simulink model "RA_Modes"  (R2022b)
settings: Solver=FixedStepAuto  StartTime=0.0  StopTime=10.0  FixedStep=1e-3  RelTol=1e-3  EnableMultiTasking=on
undefined symbols (not defined in the file): D0, D1, D10, D11, D12, D13, D2, D3, D4, D5, D6, D7, D8, D9, PTA0, PTA1, PTA2, PTB23, PTB9, PTC16, PTC17, PTC2, PTC3, PTC4, PTD0, PTD1, PTD2, PTD3
libraries: frdmk64flib x18, dspstat3 x1
settings Model: ExtModeTrigDuration=5  Creator=sarahalabdulrazzak  LastModifiedBy=kavem
settings SolverCC: AlgebraicLoopSolver=TrustRegion
settings OptimizationCC: EnhancedBackFolding=on  PassReuseOutputArgsAs=Individual arguments  ZeroExternalMemoryAtStartup=off  ZeroInternalMemoryAtStartup=off  MaxStackSize=64  OptimizeBlockOrder=speed  DifferentSizesBufferReuse=on  OptimizationCustomize=off  EfficientTunableParamExpr=on
settings DebuggingCC: ParameterTunabilityLossMsg=error  UnconnectedInputMsg=warning  UnconnectedOutputMsg=warning  UnconnectedLineMsg=warning  SFMachineParentedDataDiag=warning
settings HardwareCC: ProdBitPerPointer=32  ProdBitPerSizeT=32  ProdBitPerPtrDiffT=32  ProdLargestAtomicInteger=Long  ProdLargestAtomicFloat=Double  ProdWordSize=32  ProdHWDeviceType=ARM Compatible->ARM Cortex
settings ModelReferenceCC: EnableRefExpFcnMdlSchedulingChecks=on
settings SFSimCC: MATLABDynamicMemAlloc=off
settings RTWCC: Description=Embedded Coder  SystemTargetFile=ert.tlc  HardwareBoard=NXP FRDM-K64F  TLCOptions="-aInlineSetEventsForThisBaseRateFcn=TLC_FALSE -aSuppressMultiTaskScheduler=TLC_FALSE  -aRateBasedStepFcn=0"  TemplateMakefile=ert_default_tmf  Toolchain=GNU Tools for ARM Embedded Processors
settings CodeAppCC: ForceParamTrailComments=on  IgnoreCustomStorageClasses=off  OperatorAnnotations=on  SimulinkDataObjDesc=on  SFDataObjDesc=on  InsertBlockDesc=on

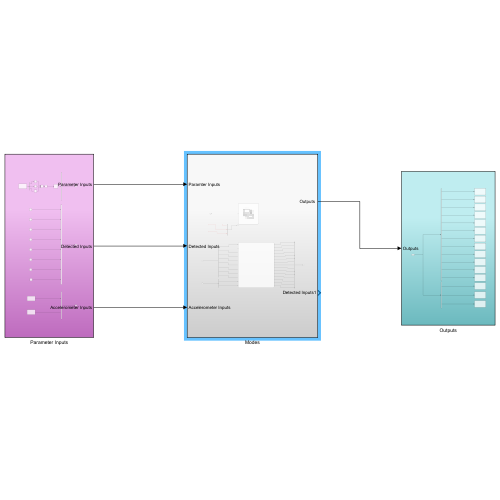
[thumbnail: Simulink's stored preview of the top-level diagram]
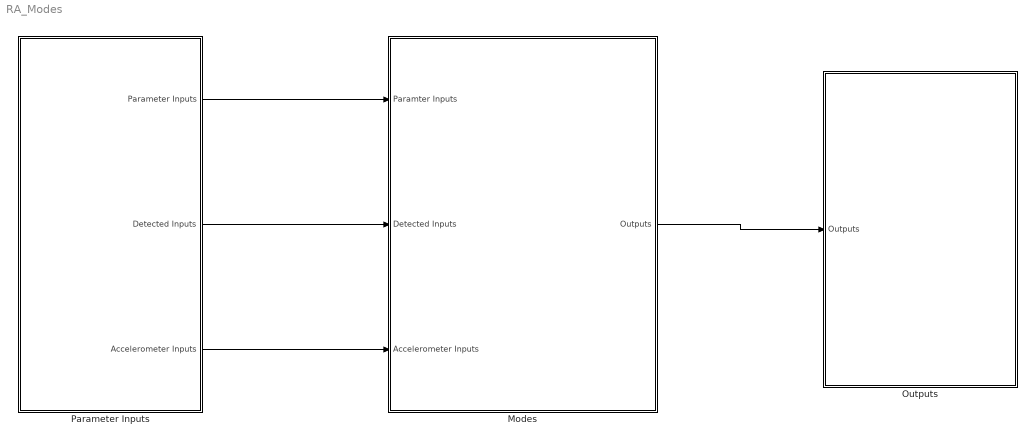
== system RA_Modes ==
  Modes : Subsystem
  Outputs : Subsystem
  Parameter Inputs : Subsystem
  wires:
  Parameter Inputs/1(Parameter Inputs) -> Modes/1(Paramter Inputs)
  Parameter Inputs/2(Detected Inputs) -> Modes/2(Detected Inputs)
  Modes/1("Outputs ") -> Outputs/1("Outputs ")
  Parameter Inputs/3(Accelerometer Inputs) -> Modes/3(Accelerometer Inputs)

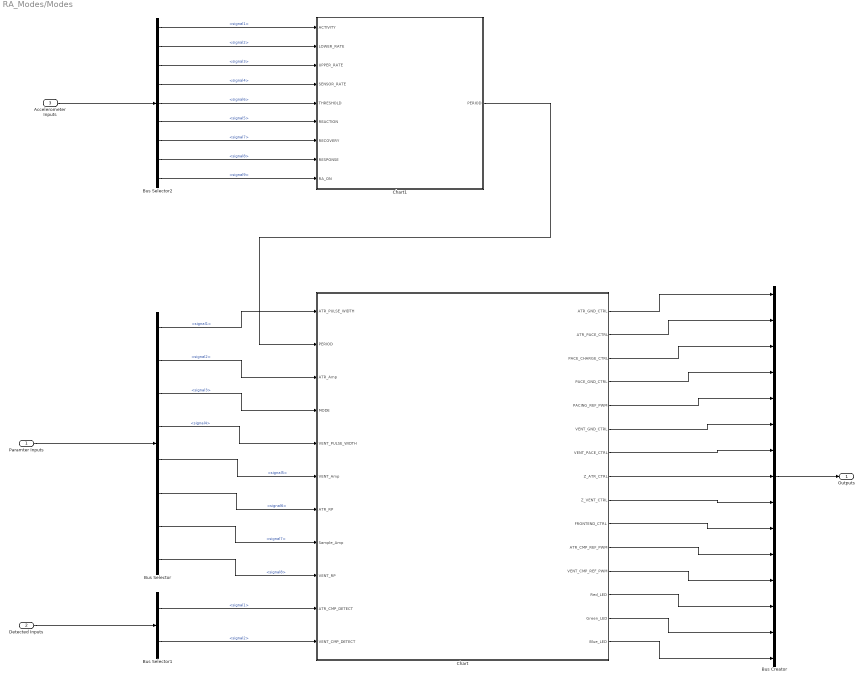
== system RA_Modes/Modes ==
  Paramter Inputs : Inport
  Detected Inputs : Inport  Port=2
  Accelerometer Inputs : Inport  Port=3
  Bus Creator : BusCreator  Inputs=15
  Bus Selector : BusSelector  OutputSignals=signal1,signal2,signal3,signal4,signal5,signal6,signal7,signal8
  Bus Selector1 : BusSelector  OutputSignals=signal1,signal2
  Bus Selector2 : BusSelector  OutputSignals=signal1,signal2,signal3,signal4,signal6,signal5,signal7,signal8,signal9
  Chart : Stateflow chart  TreatAsAtomicUnit=on
  Chart1 : Stateflow chart  TreatAsAtomicUnit=on
  "Outputs " : Outport
  wires:
  Paramter Inputs/1 -> Bus Selector/1
  Detected Inputs/1 -> Bus Selector1/1
  Bus Selector/1 -> Chart/1(ATR_PULSE_WIDTH)  "<signal1>"
  Chart/1(ATR_GND_CTRL) -> Bus Creator/1
  Chart/2(ATR_PACE_CTRL) -> Bus Creator/2
  Chart/4(PACE_GND_CTRL) -> Bus Creator/4
  Chart/5(PACING_REF_PWM) -> Bus Creator/5
  Chart/6(VENT_GND_CTRL) -> Bus Creator/6
  Chart/7(VENT_PACE_CTRL) -> Bus Creator/7
  Chart/8(Z_ATR_CTRL) -> Bus Creator/8
  Chart/9(Z_VENT_CTRL) -> Bus Creator/9
  Chart/10(FRONTEND_CTRL) -> Bus Creator/10
  Chart/11(ATR_CMP_REF_PWM) -> Bus Creator/11
  Chart/12(VENT_CMP_REF_PWM) -> Bus Creator/12
  Bus Creator/1 -> "Outputs "/1
  Chart/14(Green_LED) -> Bus Creator/14
  Chart/15(Blue_LED) -> Bus Creator/15
  Bus Selector1/1 -> Chart/10(ATR_CMP_DETECT)  "<signal1>"
  Bus Selector1/2 -> Chart/11(VENT_CMP_DETECT)  "<signal2>"
  Chart/3(PACE_CHARGE_CTRL) -> Bus Creator/3
  Chart/13(Red_LED) -> Bus Creator/13
  Bus Selector/2 -> Chart/3(ATR_Amp)  "<signal2>"
  Bus Selector/3 -> Chart/4(MODE)  "<signal3>"
  Bus Selector/4 -> Chart/5(VENT_PULSE_WIDTH)  "<signal4>"
  Bus Selector/5 -> Chart/6(VENT_Amp)  "<signal5>"
  Bus Selector/6 -> Chart/7(ATR_RP)  "<signal6>"
  Bus Selector/7 -> Chart/8(Sample_Amp)  "<signal7>"
  Bus Selector/8 -> Chart/9(VENT_RP)  "<signal8>"
  Accelerometer Inputs/1 -> Bus Selector2/1
  Bus Selector2/1 -> Chart1/1(ACTIVITY)  "<signal1>"
  Bus Selector2/2 -> Chart1/2(LOWER_RATE)  "<signal2>"
  Bus Selector2/3 -> Chart1/3(UPPER_RATE)  "<signal3>"
  Bus Selector2/4 -> Chart1/4(SENSOR_RATE)  "<signal4>"
  Bus Selector2/5 -> Chart1/5(THRESHOLD)  "<signal6>"
  Bus Selector2/6 -> Chart1/6(REACTION)  "<signal5>"
  Bus Selector2/7 -> Chart1/7(RECOVERY)  "<signal7>"
  Bus Selector2/8 -> Chart1/8(RESPONSE)  "<signal8>"
  Bus Selector2/9 -> Chart1/9(RA_ON)  "<signal9>"
  Chart1/1(PERIOD) -> Chart/2(PERIOD)

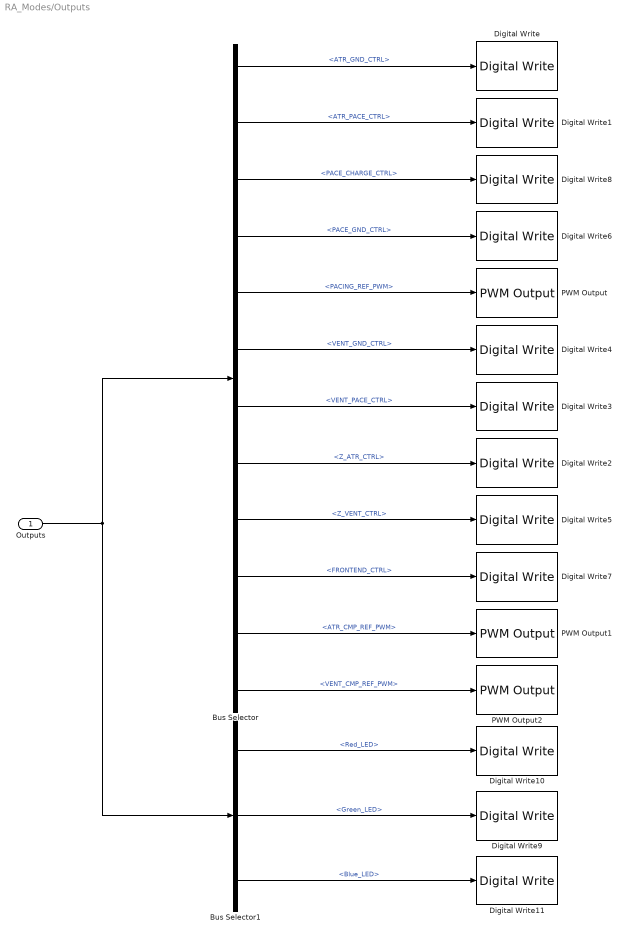
== system RA_Modes/Outputs ==
  "Outputs " : Inport
  Bus Selector : BusSelector  OutputSignals=ATR_GND_CTRL,ATR_PACE_CTRL,PACE_CHARGE_CTRL,PACE_GND_CTRL,PACING_REF_PWM,VENT_GND_CTRL,VENT_PACE_CTRL,Z_ATR_CTRL,Z_VENT_CTRL,FRONTEND_CTRL,ATR_CMP_REF_PWM,VENT_CMP_REF_PWM
  Bus Selector1 : BusSelector  OutputSignals=Red_LED,Green_LED,Blue_LED
  Digital Write : frdmk64flib/Digital Write  Whichpin=PTD2 (D11)
  Digital Write1 : frdmk64flib/Digital Write  Whichpin=PTA0 (D8)
  Digital Write10 : frdmk64flib/Digital Write  Whichpin=RED_LED
  Digital Write11 : frdmk64flib/Digital Write  Whichpin=BLUE_LED
  Digital Write2 : frdmk64flib/Digital Write  Whichpin=PTB23 (D4)
  Digital Write3 : frdmk64flib/Digital Write  Whichpin=PTC4 (D9)
  Digital Write4 : frdmk64flib/Digital Write  Whichpin=PTD3 (D12)
  Digital Write5 : frdmk64flib/Digital Write  Whichpin=PTC3 (D7)
  Digital Write6 : frdmk64flib/Digital Write  Whichpin=PTD0 (D10)
  Digital Write7 : frdmk64flib/Digital Write  Whichpin=PTD1 (D13)
  Digital Write8 : frdmk64flib/Digital Write  Whichpin=PTB9 (D2)
  Digital Write9 : frdmk64flib/Digital Write  Whichpin=GREEN_LED
  PWM Output : frdmk64flib/PWM Output  Whichpin=PTA2 (D5)  InitialFrequency=2000  InitialDutyCycle=0
  PWM Output1 : frdmk64flib/PWM Output  Whichpin=PTC2 (D6)  InitialFrequency=2000  InitialDutyCycle=0
  PWM Output2 : frdmk64flib/PWM Output  Whichpin=PTA1 (D3)  InitialFrequency=2000  InitialDutyCycle=0
  wires:
  Bus Selector/1 -> Digital Write/1  "<ATR_GND_CTRL>"
  Bus Selector/2 -> Digital Write1/1  "<ATR_PACE_CTRL>"
  Bus Selector/3 -> Digital Write8/1  "<PACE_CHARGE_CTRL>"
  Bus Selector/4 -> Digital Write6/1  "<PACE_GND_CTRL>"
  Bus Selector/5 -> PWM Output/1  "<PACING_REF_PWM>"
  Bus Selector/6 -> Digital Write4/1  "<VENT_GND_CTRL>"
  Bus Selector/7 -> Digital Write3/1  "<VENT_PACE_CTRL>"
  Bus Selector/8 -> Digital Write2/1  "<Z_ATR_CTRL>"
  Bus Selector/9 -> Digital Write5/1  "<Z_VENT_CTRL>"
  Bus Selector/10 -> Digital Write7/1  "<FRONTEND_CTRL>"
  Bus Selector/11 -> PWM Output1/1  "<ATR_CMP_REF_PWM>"
  Bus Selector/12 -> PWM Output2/1  "<VENT_CMP_REF_PWM>"
  "Outputs "/1 -> Bus Selector/1, Bus Selector1/1
  Bus Selector1/1 -> Digital Write10/1  "<Red_LED>"
  Bus Selector1/2 -> Digital Write9/1  "<Green_LED>"
  Bus Selector1/3 -> Digital Write11/1  "<Blue_LED>"

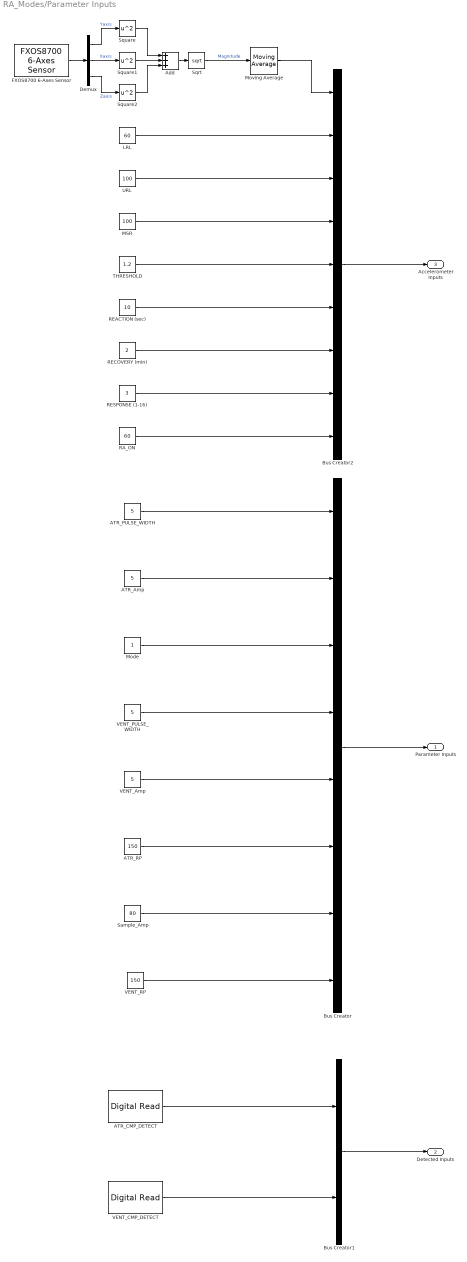
== system RA_Modes/Parameter Inputs ==
  ATR_Amp : Constant  Value=5
  ATR_CMP_DETECT : frdmk64flib/Digital Read  Whichpin=PTC16 (D0)  SampleTime=-1
  ATR_PULSE_WIDTH : Constant  Value=5
  ATR_RP : Constant  Value=150
  Add : Sum  Inputs=+++
  Bus Creator : BusCreator  Inputs=8
  Bus Creator1 : BusCreator  Inputs=2
  Bus Creator2 : BusCreator  Inputs=9
  Demux : Demux  Outputs=3
  FXOS8700 6-Axes Sensor : frdmk64flib/FXOS8700 6-Axes Sensor  Activesensor=Accelerometer only  ODR=800Hz  HybridODR=400Hz  Accelfullrange=-4g to +4g  SampleTime=-1
  LRL : Constant  Value=60
  MSR : Constant  Value=100
  Mode : Constant
  Moving Average : dspstat3/Moving Average  Method=Exponential weighting  ForgettingFactorPort=off  SpecifyWindowLength=on  WindowLength=4  OverlapLength=3  AllowArbitraryInputLength=off  ForgettingFactor=0.999  SimulateUsing=Code generation
  RA_ON : Constant  Value=60
  REACTION (sec) : Constant  Value=10
  RECOVERY (min) : Constant  Value=2
  RESPONSE (1-16) : Constant  Value=3
  Sample_Amp : Constant  Value=80
  Sqrt : Sqrt
  Square : Math  Operator=square
  Square1 : Math  Operator=square
  Square2 : Math  Operator=square
  THRESHOLD : Constant  Value=1.2
  URL : Constant  Value=100
  VENT_Amp : Constant  Value=5
  VENT_CMP_DETECT : frdmk64flib/Digital Read  Whichpin=PTC17 (D1)  SampleTime=-1
  VENT_PULSE_WIDTH : Constant  Value=5
  VENT_RP : Constant  Value=150
  Parameter Inputs : Outport
  Detected Inputs : Outport  Port=2
  Accelerometer Inputs : Outport  Port=3
  wires:
  Bus Creator/1 -> Parameter Inputs/1
  ATR_PULSE_WIDTH/1 -> Bus Creator/1
  ATR_Amp/1 -> Bus Creator/2
  Mode/1 -> Bus Creator/3
  VENT_PULSE_WIDTH/1 -> Bus Creator/4
  VENT_Amp/1 -> Bus Creator/5
  ATR_RP/1 -> Bus Creator/6
  Sample_Amp/1 -> Bus Creator/7
  VENT_RP/1 -> Bus Creator/8
  Bus Creator1/1 -> Detected Inputs/1
  VENT_CMP_DETECT/1 -> Bus Creator1/2
  ATR_CMP_DETECT/1 -> Bus Creator1/1
  Sqrt/1 -> Moving Average/1  "Magnitude"
  Demux/3 -> Square2/1  "Zaxis"
  Square2/1 -> Add/3
  Add/1 -> Sqrt/1
  Demux/2 -> Square1/1  "Xaxis"
  Square/1 -> Add/1
  Demux/1 -> Square/1  "Yaxis"
  FXOS8700 6-Axes Sensor/1 -> Demux/1
  Square1/1 -> Add/2
  Bus Creator2/1 -> Accelerometer Inputs/1
  Moving Average/1 -> Bus Creator2/1
  LRL/1 -> Bus Creator2/2
  URL/1 -> Bus Creator2/3
  MSR/1 -> Bus Creator2/4
  RA_ON/1 -> Bus Creator2/9
  REACTION (sec)/1 -> Bus Creator2/6
  THRESHOLD/1 -> Bus Creator2/5
  RECOVERY (min)/1 -> Bus Creator2/7
  RESPONSE (1-16)/1 -> Bus Creator2/8

== stateflow chart RA_Modes/Modes/Chart ==
  state Identify_Mode_Path
    entry:
    % MODE = 1 (AOO)
    % MODE = 2 (AAI)
    % MODE = 3 (VOO)
    % MODE = 4 (VVI)
    %
    %pacemaker disconnected
    %stop sensing
    PACE_CHARGE_CTRL = LOW
    VENT_PACE_CTRL = LOW
    ATR_PACE_CTRL = LOW
    PACE_GND_CTRL = LOW
    ATR_GND_CTRL = LOW
    VENT_GND_CTRL = LOW
    Z_ATR_CTRL = LOW
    Z_VENT_CTRL = LOW
    FRONTEND_CTRL = LOW
  state AOO
    entry:
    %Charge primary capcitor C22
    ATR_PACE_CTRL=LOW
    PACING_REF_PWM = 20*ATR_Amp
    PACE_CHARGE_CTRL = HIGH
    %Discharge block capacitor C21
    PACE_GND_CTRL = HIGH
    ATR_GND_CTRL = HIGH
    %use LED  to verify state
    Red_LED=false
    Green_LED=false
    Blue_LED=false
  state AOO_ATR_PULSE
    entry:
    %Discharge C22 primary capacitor
    %Charge C21 block capacitor
    PACE_CHARGE_CTRL = LOW
    PACE_GND_CTRL = HIGH
    ATR_PACE_CTRL = HIGH
    ATR_GND_CTRL = LOW
    PACING_REF_PWM = 20*ATR_Amp
    %use LED  to verify state
    Red_LED=true
    Green_LED=false
    Blue_LED=false
  state AAI
    entry:
    %sensing ON
    FRONTEND_CTRL = HIGH
    %Charge primary capcitor C22
    ATR_PACE_CTRL=LOW
    PACING_REF_PWM = 20*ATR_Amp
    PACE_CHARGE_CTRL = HIGH
    %Discharge block capacitor C21
    PACE_GND_CTRL = HIGH
    ATR_GND_CTRL = HIGH
    ATR_CMP_REF_PWM = Sample_Amp
    %use LED  to verify state
    Red_LED=false
    Blue_LED=false
    Green_LED=false
  state AAI_ATR_PULSE
    entry:
    %sensing OFF
    FRONTEND_CTRL = LOW
    %Discharge C22 primary capacitor
    %Charge C21 block capacitor
    PACE_CHARGE_CTRL = LOW
    PACE_GND_CTRL = HIGH
    ATR_PACE_CTRL = HIGH
    ATR_GND_CTRL = LOW
    PACING_REF_PWM = 20*ATR_Amp
    %use LED  to verify state
    Red_LED=false
    Green_LED=false
    Blue_LED=true
  state VOO
    entry:
    %Charge primary capcitor C22
    VENT_PACE_CTRL=LOW
    PACING_REF_PWM = 20*VENT_Amp
    PACE_CHARGE_CTRL = HIGH
    %Discharge block capacitor C21
    PACE_GND_CTRL = HIGH
    VENT_GND_CTRL = HIGH
    %use LED  to verify state
    Red_LED=false
    Green_LED=false
    Blue_LED=false
  state VOO_VENT_PULSE
    entry:
    %Discharge C22 primary capacitor
    %Charge C21 block capacitor
    PACE_CHARGE_CTRL = LOW
    PACE_GND_CTRL = HIGH
    VENT_GND_CTRL = LOW
    VENT_PACE_CTRL  = HIGH
    PACING_REF_PWM = 20*VENT_Amp
    %use LED  to verify state
    Red_LED=false
    Green_LED=true
    Blue_LED=false
  state VVI
    entry:
    %sensing ON
    FRONTEND_CTRL = HIGH
    %Charge primary capcitor C22
    VENT_PACE_CTRL= LOW
    PACING_REF_PWM = 20*VENT_Amp
    PACE_CHARGE_CTRL = HIGH
    %Discharge block capacitor C21
    PACE_GND_CTRL = HIGH
    VENT_PACE_CTRL = LOW
    VENT_GND_CTRL = HIGH
    VENT_CMP_REF_PWM = Sample_Amp
    %use LED  to verify state
    Red_LED=true
    Green_LED=false
    Blue_LED=false
  state VVI_VENT_PULSE
    %sensing OFF
    FRONTEND_CTRL = LOW
    %Discharge C22 primary capacitor
    %Charge C21 block capacitor
    PACE_CHARGE_CTRL = LOW
    PACE_GND_CTRL = HIGH
    VENT_GND_CTRL = LOW
    VENT_PACE_CTRL  = HIGH
    PACING_REF_PWM = 20*VENT_Amp
    %use LED  to verify state
    Red_LED=false
    Green_LED=true
    Blue_LED=false
  (default) -> Identify_Mode_Path
  AOO -> AOO_ATR_PULSE : after(PERIOD - ATR_PULSE_WIDTH,msec)
  Identify_Mode_Path -> AOO [order 1] : [MODE == 1]
  AOO_ATR_PULSE -> AOO : after(ATR_PULSE_WIDTH,msec)
  AAI_ATR_PULSE -> AAI : after(ATR_PULSE_WIDTH,msec)
  Identify_Mode_Path -> AAI [order 2] : [MODE == 2]
  AAI -> (junction 41)
  (junction 41) -> AAI_ATR_PULSE [order 1] : after(PERIOD - ATR_PULSE_WIDTH,msec)[ATR_CMP_DETECT == LOW]
  (junction 41) -> AAI [order 2] : after(ATR_RP, msec)[ATR_CMP_DETECT == HIGH]
  VOO -> VOO_VENT_PULSE : after(PERIOD - VENT_PULSE_WIDTH,msec)
  Identify_Mode_Path -> VOO [order 3] : [MODE == 3]
  VOO_VENT_PULSE -> VOO : after(VENT_PULSE_WIDTH,msec)
  VVI_VENT_PULSE -> VVI : after(VENT_PULSE_WIDTH,msec)
  Identify_Mode_Path -> VVI [order 4] : [MODE == 4]
  VVI -> (junction 61)
  (junction 61) -> VVI_VENT_PULSE [order 1] : after(PERIOD - VENT_PULSE_WIDTH,msec)[VENT_CMP_DETECT == LOW]
  (junction 61) -> VVI [order 2] : after(VENT_RP, msec)[VENT_CMP_DETECT == HIGH]
  data: ATR_PULSE_WIDTH input; PERIOD input; ATR_Amp input; MODE input; VENT_PULSE_WIDTH input; VENT_Amp input; ATR_RP input; Sample_Amp input; VENT_RP input; ATR_CMP_DETECT input; VENT_CMP_DETECT input; HIGH local =1; LOW local =0; ATR_GND_CTRL output; ATR_PACE_CTRL output; PACE_CHARGE_CTRL output; PACE_GND_CTRL output; PACING_REF_PWM output; VENT_GND_CTRL output; VENT_PACE_CTRL output; Z_ATR_CTRL output; Z_VENT_CTRL output; FRONTEND_CTRL output; ATR_CMP_REF_PWM output; VENT_CMP_REF_PWM output; Red_LED output; Green_LED output; Blue_LED output

== stateflow chart RA_Modes/Modes/Chart1 ==
  state RECOVER_RATE
    %this is for if the RA is turned off while the
    %slowly shift activity (might not need)
    %if the period is above LRL, reduce by amount that will bring diff to 0 within recovery time
    AVG_ACT = (AVG_ACT+ACTIVITY)/2
    if PERIOD > LOWER_RATE
    PERIOD = PERIOD - (SENSOR_RATE-LOWER_RATE)/(RECOVERY*1000)
    DELAY = (RECOVERY*1000)
    else
    PERIOD = LOWER_RATE
    DELAY = 0
    end
  state RA_OFF
    %set the period to LRL
    %read current activity
    %and assign to var.
    entry:
    PERIOD = LOWER_RATE
    AVG_ACT = ACTIVITY
    if SENSOR_RATE > UPPER_RATE
    SENSOR_RATE = UPPER_RATE
    end
  state SET_TARGET
    %set the target rate and make sure it falls within the bounds
    TARGET_RATE = (RESPONSE^2-RESPONSE+30)*(AVG_ACT*THRESHOLD)+LOWER_RATE
    if TARGET_RATE > SENSOR_RATE
    TARGET_RATE = SENSOR_RATE
    elseif TARGET_RATE < LOWER_RATE
    TARGET_RATE = LOWER_RATE
    end
  state RA_ON
  state RECOVER_REACT
    %slowly shift activity (might not need)
    %if Period is above target, decrease using recovery
    %if below target, increase using reaction
    AVG_ACT = (AVG_ACT+ACTIVITY)/2
    if PERIOD > TARGET_RATE
    PERIOD = PERIOD - (SENSOR_RATE-LOWER_RATE)/(RECOVERY*1000)
    DELAY = (RECOVERY*1000)
    elseif PERIOD < TARGET_RATE
    PERIOD = PERIOD + (SENSOR_RATE-LOWER_RATE)/(REACTION*100)
    DELAY = (REACTION*100)
    end
  RECOVER_RATE -> SET_TARGET [order 1] : [n >= DELAY && AVG_ACT >= THRESHOLD]
  RECOVER_RATE -> RECOVER_RATE [order 2] : after(1,msec){n = n+1}
  RECOVER_RATE -> RA_OFF [order 3] : [RA_ON == FALSE && n >= DELAY]
  RA_ON -> RECOVER_RATE [order 1] : [AVG_ACT < THRESHOLD]{n=0}
  (default) -> RA_OFF
  RA_ON -> SET_TARGET [order 2] : [AVG_ACT >= THRESHOLD]
  RA_OFF -> RA_ON : [RA_ON == TRUE]{TARGET_RATE=PERIOD}
  RECOVER_REACT -> RA_ON [order 1] : [n >= DELAY]
  SET_TARGET -> RECOVER_REACT : {n = 0, AVG_ACT = ACTIVITY}
  RECOVER_REACT -> RECOVER_REACT [order 2] : after(1,msec){n = n+1}
  data: ACTIVITY input; LOWER_RATE input; UPPER_RATE input; SENSOR_RATE input; THRESHOLD input; REACTION input; RECOVERY input; RESPONSE input; RA_ON input; PERIOD output; TRUE local =1; FALSE local =0; TARGET_RATE local; AVG_ACT local; DELAY local; n local
